simulink model "dinamica_corpo_3d_ML2013a_simulacao"  (R2013a)
settings: Solver=ode45  StartTime=0.0  StopTime=500  RelTol=1e-3
libraries: aerolibutil x2, vrlib x2, aerolibtransform2 x1
settings Model: Creator=Daniel  LastModifiedBy=Daniel

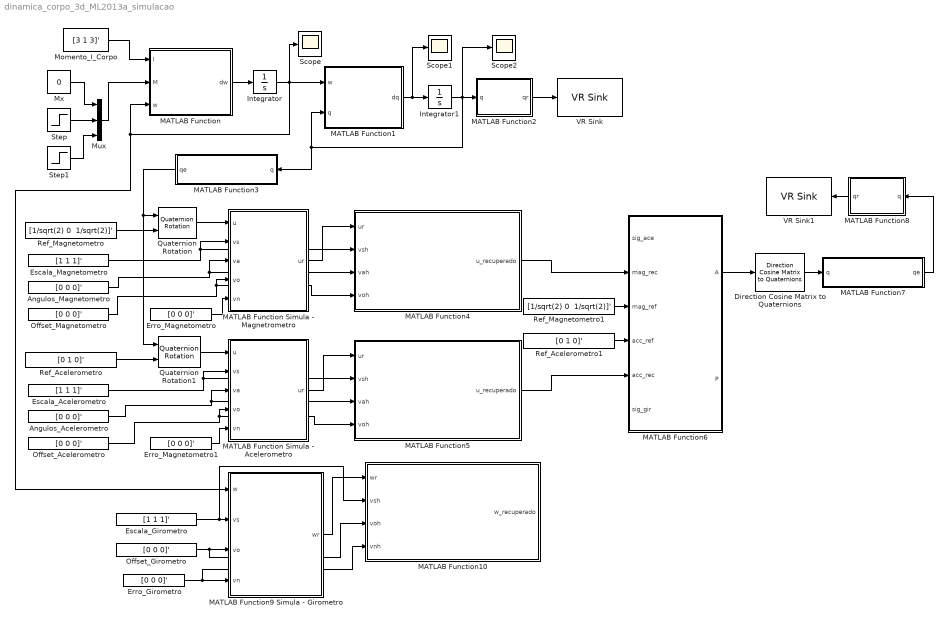
== system dinamica_corpo_3d_ML2013a_simulacao ==
  Angulos_Acelerometro : Constant  Value=[0 0 0]'
  Angulos_Magnetometro : Constant  Value=[0 0 0]'
  Direction Cosine Matrix to Quaternions : aerolibtransform2/Direction Cosine Matrix  to Quaternions
  Erro_Girometro : Constant  Value=[0 0 0]'
  Erro_Magnetometro : Constant  Value=[0 0 0]'
  Erro_Magnetometro1 : Constant  Value=[0 0 0]'
  Escala_Acelerometro : Constant  Value=[1 1 1]'
  Escala_Girometro : Constant  Value=[1 1 1]'
  Escala_Magnetometro : Constant  Value=[1 1 1]'
  Integrator : Integrator  InitialCondition=[0 0 0]
  Integrator1 : Integrator  InitialCondition=[1 0 0 0]
  MATLAB Function : MATLAB Function  TreatAsAtomicUnit=on
  MATLAB Function Simula - Acelerometro : MATLAB Function  TreatAsAtomicUnit=on
  MATLAB Function Simula - Magnetrometro : MATLAB Function  TreatAsAtomicUnit=on
  MATLAB Function1 : MATLAB Function  TreatAsAtomicUnit=on
  MATLAB Function10 : MATLAB Function  TreatAsAtomicUnit=on
  MATLAB Function2 : MATLAB Function  TreatAsAtomicUnit=on
  MATLAB Function3 : MATLAB Function  TreatAsAtomicUnit=on
  MATLAB Function4 : MATLAB Function  TreatAsAtomicUnit=on
  MATLAB Function5 : MATLAB Function  TreatAsAtomicUnit=on
  MATLAB Function6 : MATLAB Function  TreatAsAtomicUnit=on
  MATLAB Function7 : MATLAB Function  TreatAsAtomicUnit=on
  MATLAB Function8 : MATLAB Function  TreatAsAtomicUnit=on
  MATLAB Function9 Simula - Girometro : MATLAB Function  TreatAsAtomicUnit=on
  Momento_I_Corpo : Constant  Value=[3 1 3]'
  Mux : Mux  Inputs=3
  Mx : Constant  Value=0
  Offset_Acelerometro : Constant  Value=[0 0 0]'
  Offset_Girometro : Constant  Value=[0 0 0]'
  Offset_Magnetometro : Constant  Value=[0 0 0]'
  Quaternion Rotation : aerolibutil/Quaternion Rotation
  Quaternion Rotation1 : aerolibutil/Quaternion Rotation
  Ref_Acelerometro : Constant  Value=[0 1 0]'
  Ref_Acelerometro1 : Constant  Value=[0 1 0]'
  Ref_Magnetometro : Constant  Value="[1/sqrt(2) 0  1/sqrt(2)]'"
  Ref_Magnetometro1 : Constant  Value="[1/sqrt(2) 0  1/sqrt(2)]'"
  Scope : Scope
  Scope1 : Scope
  Scope2 : Scope
      settings: SaveName=ScopeData2
  Step : Step  Before=1  After=0  SampleTime=0
  Step1 : Step  Before=.2  After=0  SampleTime=0
  VR Sink : vrlib/VR Sink  InstantiateOnLoad=on  SampleTime=-1  ViewEnable=on  RemoteChange=off  RemoteView=off  FieldsWritten=H.rotation.4.1.1.double  WorldFileName=C:\Users\Daniel\Desktop\TCC Daniel\Arquivos WRL\cilindro1_2013.wrl  AutoView=off  VideoDimensions=[]  AllowVariableSize=off
  VR Sink1 : vrlib/VR Sink  InstantiateOnLoad=on  SampleTime=-1  ViewEnable=on  RemoteChange=off  RemoteView=off  FieldsWritten=H.rotation.4.1.1.double  WorldFileName=C:\Users\Daniel\Desktop\TCC Daniel\Arquivos WRL\cilindro2_2013.wrl  AutoView=off  VideoDimensions=[]  AllowVariableSize=off
  wires:
  Momento_I_Corpo/1 -> MATLAB Function/1(I)
  Mux/1 -> MATLAB Function/2(M)
  Mx/1 -> Mux/1
  Step/1 -> Mux/2
  Step1/1 -> Mux/3
  MATLAB Function/1(dw) -> Integrator/1
  Integrator/1 -> MATLAB Function1/1(w), Scope/1, MATLAB Function/3(w), MATLAB Function9 Simula - Girometro/1(w)
  MATLAB Function1/1(dq) -> Integrator1/1, Scope1/1
  Integrator1/1 -> MATLAB Function3/1(q), MATLAB Function1/2(q), Scope2/1, MATLAB Function2/1(q)
  MATLAB Function2/1(qr) -> VR Sink/1
  Quaternion Rotation/1 -> MATLAB Function Simula - Magnetrometro/1(u)
  Quaternion Rotation1/1 -> MATLAB Function Simula - Acelerometro/1(u)
  MATLAB Function3/1(qe) -> Quaternion Rotation/1, Quaternion Rotation1/1
  Ref_Magnetometro/1 -> Quaternion Rotation/2
  Ref_Acelerometro/1 -> Quaternion Rotation1/2
  Erro_Magnetometro/1 -> MATLAB Function Simula - Magnetrometro/5(vn)
  Erro_Magnetometro1/1 -> MATLAB Function Simula - Acelerometro/5(vn)
  Offset_Magnetometro/1 -> MATLAB Function Simula - Magnetrometro/4(vo), MATLAB Function4/4(voh)
  Escala_Acelerometro/1 -> MATLAB Function Simula - Acelerometro/2(vs), MATLAB Function5/2(vsh)
  Angulos_Acelerometro/1 -> MATLAB Function Simula - Acelerometro/3(va), MATLAB Function5/3(vah)
  Offset_Acelerometro/1 -> MATLAB Function Simula - Acelerometro/4(vo), MATLAB Function5/4(voh)
  MATLAB Function Simula - Magnetrometro/1(ur) -> MATLAB Function4/1(ur)
  MATLAB Function Simula - Acelerometro/1(ur) -> MATLAB Function5/1(ur)
  Escala_Magnetometro/1 -> MATLAB Function Simula - Magnetrometro/2(vs), MATLAB Function4/2(vsh)
  Angulos_Magnetometro/1 -> MATLAB Function Simula - Magnetrometro/3(va), MATLAB Function4/3(vah)
  MATLAB Function5/1(u_recuperado) -> MATLAB Function6/5(acc_rec)
  MATLAB Function4/1(u_recuperado) -> MATLAB Function6/2(mag_rec)
  Ref_Magnetometro1/1 -> MATLAB Function6/3(mag_ref)
  Ref_Acelerometro1/1 -> MATLAB Function6/4(acc_ref)
  MATLAB Function6/1(A) -> Direction Cosine Matrix to Quaternions/1
  MATLAB Function7/1(qe) -> MATLAB Function8/1(q)
  MATLAB Function8/1(qr) -> VR Sink1/1
  MATLAB Function9 Simula - Girometro/1(wr) -> MATLAB Function10/1(wr)
  Escala_Girometro/1 -> MATLAB Function10/2(vsh), MATLAB Function9 Simula - Girometro/2(vs)
  Offset_Girometro/1 -> MATLAB Function10/3(voh), MATLAB Function9 Simula - Girometro/3(vo)
  Direction Cosine Matrix to Quaternions/1 -> MATLAB Function7/1(q)
  Erro_Girometro/1 -> MATLAB Function10/4(vnh), MATLAB Function9 Simula - Girometro/4(vn)

== matlab function dinamica_corpo_3d_ML2013a_simulacao/MATLAB Function1 ==
  data: w input; dq output; q input
function dq = cinematica(w,q)
%#eml
wx = w(1);
wy = w(2);
wz = w(3);

q = q/norm(q);

qteta = q(1);
qx = q(2);
qy = q(3);
qz = q(4);

W = [0 -wx -wy -wz; wx 0 wz -wy; wy -wz 0 wx; wz wy -wx 0];
%W=[0 wz -wy wx; -wz 0 wx wy; wy -wx 0 wz; -wx -wy -wz 0];
dq=0.5*W*[qteta qx qy qz]';

== matlab function dinamica_corpo_3d_ML2013a_simulacao/MATLAB Function ==
  data: I input; dw output; M input; w input
function dw  = Eq_Euler(I,M,w)
%#eml
wx = w(1);
wy = w(2);
wz = w(3);

Ix = I(1);
Iy = I(2);
Iz = I(3);

Mx = M(1);
My = M(2);
Mz = M(3);

dwx = (Mx - wy*wz*(Iz - Iy))/Ix;
dwy = (My - wx*wz*(Ix - Iz))/Iy;
dwz = (Mz - wx*wy*(Iy - Ix))/Iz;

dw=[dwx dwy dwz]';

== matlab function dinamica_corpo_3d_ML2013a_simulacao/MATLAB Function2 ==
  data: q input; qr output
function qr = ajusta_q(q)
%#eml

q = q/(norm(q));
v = [q(2) q(3) q(4)] / norm([q(2) q(3) q(4)]);
ang = acos(q(1))*2;

qr = [v ang];

== matlab function dinamica_corpo_3d_ML2013a_simulacao/MATLAB Function3 ==
  data: q input; qe output
function qe = tira_redundancia(q)
qe = zeros(4,1);
%#eml

if q(1)<0
    qe = -q;
else
    qe = q;
end

== matlab function dinamica_corpo_3d_ML2013a_simulacao/MATLAB Function Simula - Magnetrometro ==
  data: u input; ur output; vs input; va input; vo input; vn input
function ur = triad_model(u,vs,va,vo,vn)
%#eml

rho = va(1);
phi = va(2);
lambda = va(3);

S = diag(vs);
T = [1 0 0; sin(rho) cos(rho) 0;...
    sin(phi)*cos(lambda) sin(lambda)*cos(phi) cos(phi)*cos(lambda)];

ur = S*T*u + vo + vn*randn;

== matlab function dinamica_corpo_3d_ML2013a_simulacao/MATLAB Function Simula - Acelerometro ==
  data: u input; ur output; vs input; va input; vo input; vn input
function ur = triad_model(u,vs,va,vo,vn)
%#eml

rho = va(1);
phi = va(2);
lambda = va(3);

S = diag(vs);
T = [1 0 0; sin(rho) cos(rho) 0;...
    sin(phi)*cos(lambda) sin(lambda)*cos(phi) cos(phi)*cos(lambda)];

ur = S*T*u + vo + vn*randn;

== matlab function dinamica_corpo_3d_ML2013a_simulacao/MATLAB Function4 ==
  data: ur input; u_recuperado output; vsh input; vah input; voh input
function u_recuperado = inv_triad_model(ur,vsh,vah,voh)
%#eml

rho = vah(1);
phi = vah(2);
lambda = vah(3);

T_inv = [1 0 0; -tan(rho) 1/cos(rho) 0;...
    tan(rho)*tan(lambda)-tan(phi) -tan(lambda)/cos(rho) 1/(cos(lambda)*cos(phi))];
S_inv = inv(diag(vsh));

u_recuperado = T_inv*S_inv*(ur - voh);

== matlab function dinamica_corpo_3d_ML2013a_simulacao/MATLAB Function5 ==
  data: ur input; u_recuperado output; vsh input; vah input; voh input
function u_recuperado = inv_triad_model(ur,vsh,vah,voh)
%#eml

rho = vah(1);
phi = vah(2);
lambda = vah(3);

T_inv = [1 0 0; -tan(rho) 1/cos(rho) 0;...
    tan(rho)*tan(lambda)-tan(phi) -tan(lambda)/cos(rho) 1/(cos(lambda)*cos(phi))];
S_inv = inv(diag(vsh));

u_recuperado = T_inv*S_inv*(ur - voh);

== matlab function dinamica_corpo_3d_ML2013a_simulacao/MATLAB Function6 ==
  data: sig_ace input; A output; mag_rec input; mag_ref input; acc_ref input; acc_rec input; sig_gir input; P output
function [A,P] = TRIAD(sig_ace,mag_rec,mag_ref,acc_ref,acc_rec,sig_gir)

% ========== Função de Determinação de Atitude ===========
% ========== Algoritmo TRIAD ===========
% Os parâmetros de Entrada são:
% V1 : vetor de referência V1
V1 = acc_ref;
% V2 : vetor de referência V2
V2 = mag_ref;
% W1 : vetor de observação W1
W1 = acc_rec;
% W2 : vetor de observação W2
W2 = mag_rec;
% SigTo1 : desvio padrão das observação do Acelerômetro
SigTot1 = sig_ace;
% SigTo2 : desvio padrão das observação do Magnetômetro
SigTot2 = sig_gir;

% ========================================================
% Os parâmetros de Retorno são:
% A : matriz de atitude
% P : Covariância da atitude
% ========================================================
% --- Obtendo a Tríade de Referência
r1 = V1/norm(V1);
r2 = cross(V1,V2); % função do produto vetorial
r2 = r2 / norm(r2);
r3 = cross(r1,r2);
% --- Montando a Matriz de Referência
Mref = [r1 r2 r3];
% --- Obtendo a tríade de observação
s1 = W1/norm(W1);
s2 = cross(W1,W2);
s2 = s2 / norm(s2);
s3 = cross(s1,s2);
% --- Montando a Matriz de Observação
Mobs = [s1 s2 s3];
% --- Atitude pelo TRIAD
A = Mobs * Mref';
%--------------------------------------------------------------------------
% Obtendo a covariância da atitude (P = P + AP AT)
P = SigTot1^2 * eye(3) + ...
    (1/norm(cross(W1,W2)))^2 * (SigTot1^2* (W1'*W2) * (W1*W2' + W2*W1')...
    + (SigTot2^2 - SigTot1^2)*W1*W1');

%--------------------------------------------------------------------------

== matlab function dinamica_corpo_3d_ML2013a_simulacao/MATLAB Function7 ==
  data: q input; qe output
function qe = tira_redundancia(q)
qe = zeros(4,1);
%#eml

if q(1)<0
    qe = -q;
else
    qe = q;
end

== matlab function dinamica_corpo_3d_ML2013a_simulacao/MATLAB Function8 ==
  data: q input; qr output
function qr = ajusta_q(q)
%#eml

q = q/(norm(q));
v = [q(2) q(3) q(4)] / norm([q(2) q(3) q(4)]);
ang = acos(q(1))*2;

qr = [v ang];

== matlab function dinamica_corpo_3d_ML2013a_simulacao/MATLAB Function9 Simula - Girometro ==
  data: w input; wr output; vs input; vo input; vn input
function wr = gyro_model(w,vs,vo,vn)
%#eml

S = diag(vs);

wr = S*w + vo + vn*randn;

== matlab function dinamica_corpo_3d_ML2013a_simulacao/MATLAB Function10 ==
  data: wr input; w_recuperado output; vsh input; voh input; vnh input
function w_recuperado = inv_gyro_model(wr,vsh,voh,vnh)
%#eml

S_inv = inv(diag(vsh));

w_recuperado = S_inv*(wr - voh);
